simulink model "CBB_ccontrol_pspice_clasicalPI"  (R2021a)
settings: Solver=VariableStepAuto  StartTime=0.0  StopTime=1  RelTol=1e-3
undefined symbols (not defined in the file): ki, kp, L, R
libraries: pspsim x1, spsSawtoothGeneratorLib x1
settings Model: Creator=omar_  LastModifiedBy=omar_

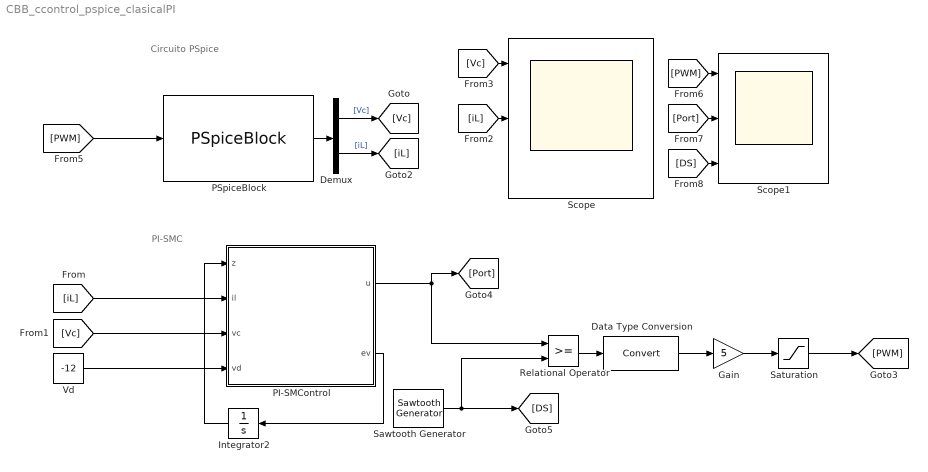
== system CBB_ccontrol_pspice_clasicalPI ==
  note: Circuito PSpice
  note: PI-SMC
  Data Type Conversion : DataTypeConversion
  Demux : Demux  Outputs=2
  Gain : Gain  Gain=5
  Integrator2 : Integrator  InitialCondition=0.001
  PI-SMControl : MATLAB Function  TreatAsAtomicUnit=on
  PSpiceBlock : pspsim/PSpiceBlock  SFunctionModules=''
      settings: SourceProductName=PSpice Block
  Relational Operator : RelationalOperator  OutDataTypeStr=boolean  RndMeth=Simplest
  Saturation : Saturate  UpperLimit=5  LowerLimit=0
  Sawtooth Generator : spsSawtoothGeneratorLib/Sawtooth Generator  Freq=50000  Phase=0  Ts=0
  Scope : Scope  NumInputPorts=3
  Scope1 : Scope  NumInputPorts=3
  Vd : Constant  Value=-12
  wires:
  [PWM] -> PSpiceBlock/1
  [DS] -> Scope1/3
  Relational Operator/1 -> Data Type Conversion/1
  [Port] -> Scope1/2
  [iL] -> PI-SMControl/2(il)
  Gain/1 -> Saturation/1
  [iL] -> Scope/2
  Integrator2/1 -> PI-SMControl/1(z)
  PSpiceBlock/1 -> Demux/1
  [Vc] -> Scope/1
  Data Type Conversion/1 -> Gain/1
  Saturation/1 -> [PWM]
  PI-SMControl/1(u) -> [Port], Relational Operator/1
  [Vc] -> PI-SMControl/3(vc)
  Demux/2 -> [iL]  "[iL]"
  Demux/1 -> [Vc]  "[Vc]"
  Sawtooth Generator/1 -> [DS], Relational Operator/2
  Vd/1 -> PI-SMControl/4(vd)
  PI-SMControl/2(ev) -> Integrator2/1
  [PWM] -> Scope1/1

== matlab function CBB_ccontrol_pspice_clasicalPI/PI-SMControl ==
  data: E parameter; u output; ki parameter; R parameter; kp parameter; z input; il input; vc input; L parameter; vd input; ev output
function [u,ev] = fcn(E, ki, R, kp, z,il,vc,L, vd)

%il = double(il); 
vc = double(vc); 
ev = double(vc -vd);
u=kp*ev+ki*z;
